simulink model "actividad3"  (R2021a)
settings: Solver=VariableStepAuto  StartTime=0.0  StopTime=2  FixedStep=1e-5  RelTol=1e-3
libraries: pid_lib x1
settings Model: Creator=Agus  LastModifiedBy=valen

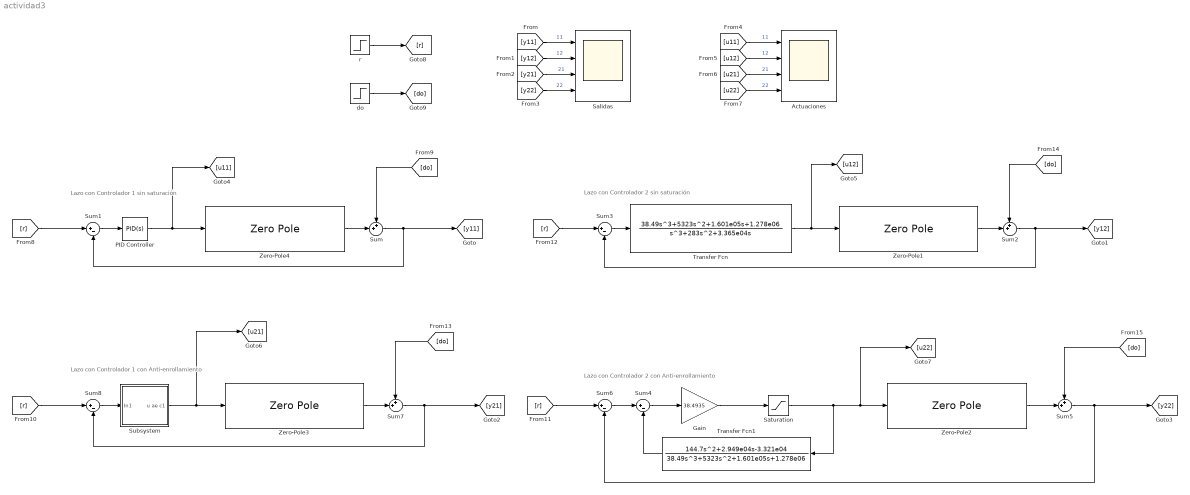
== system actividad3 ==
  note: Lazo con Controlador 1 con Anti-enrollamiento
  note: Lazo con Controlador 2 con Anti-enrollamiento
  note: Lazo con Controlador 1 sin saturación
  note: Lazo con Controlador 2 sin saturación
  Actuaciones : Scope  NumInputPorts=4
  Gain : Gain  Gain=38.4935
  PID Controller : pid_lib/PID Controller  Controller=PID  Form=Parallel  TimeDomain=Continuous-time  UseExternalTs=off  SampleTime=-1  IntegratorMethod=Forward Euler  FilterMethod=Forward Euler  ControllerParametersSource=internal  P=2.1595  I=8.175  D=0.0733  UseFilter=on  N=1364.25  TunerSelectOption=Transfer Function Based (PID Tuner App)  InitialConditionSource=internal  InitialConditionForIntegrator=0  InitialConditionForFilter=0  DifferentiatorICPrevScaledInput=0  ExternalReset=none  TrackingMode=off  Kt=1  LimitOutput=off  SatLimitsSource=internal  UpperSaturationLimit=inf  LowerSaturationLimit=-inf  LinearizeAsGain=on  AntiWindupMode=none  Kb=1  POutMin=[]  POutMax=[]  IOutMin=[]  IOutMax=[]  DOutMin=[]  DOutMax=[]  NOutMin=[]  NOutMax=[]  SumOutMin=[]  SumOutMax=[]  SaturationOutMin=[]  SaturationOutMax=[]  PParamMin=[]  PParamMax=[]  IParamMin=[]  IParamMax=[]  DParamMin=[]  DParamMax=[]  NParamMin=[]  NParamMax=[]  KbParamMin=[]  KbParamMax=[]  KtParamMin=[]  KtParamMax=[]  KbOutMin=[]  KbOutMax=[]  KtOutMin=[]  KtOutMax=[]  IntegratorOutMin=[]  IntegratorOutMax=[]  FilterOutMin=[]  FilterOutMax=[]  SumI1OutMin=[]  SumI1OutMax=[]  SumI2OutMin=[]  SumI2OutMax=[]  SumI3OutMin=[]  SumI3OutMax=[]  SumI4OutMin=[]  SumI4OutMax=[]  SumDOutMin=[]  SumDOutMax=[]  DifferentiatorOutMin=[]  DifferentiatorOutMax=[]  FilterDiffOutCoefMin=[]  FilterDiffOutCoefMax=[]  ReciprocalOutMin=[]  ReciprocalOutMax=[]  SumDenOutMin=[]  SumDenOutMax=[]  SumNumOutMin=[]  SumNumOutMax=[]  DivideOutMin=[]  DivideOutMax=[]  UdiffTsProdOutMin=[]  UdiffTsProdOutMax=[]  NTsProdOutMin=[]  NTsProdOutMax=[]  UintegralTsProdOutMin=[]  UintegralTsProdOutMax=[]  UngainTsProdOutMin=[]  UngainTsProdOutMax=[]  IntegratorContinuousStateAttributes=''  IntegratorStateMustResolveToSignalObject=off  IntegratorRTWStateStorageClass=Auto  FilterContinuousStateAttributes=''  FilterStateMustResolveToSignalObject=off  FilterRTWStateStorageClass=Auto  ParallelPVariant=InternalParameters  IdealPVariant=Disabled  IVariant=InternalParameters  DVariant=InternalParameters  IntegratorVariant=Continuous  SatVariant=Disabled  AWVariant=Passthrough  PCopyVariant=Disabled  TRVariant=Disabled  FdbkBlocksVariant=Forward  IdealPFdbkVariant=Disabled  SatFdbkVariant=Disabled  DerivativeFilterVariant=ContFilter  NVariant=InternalParameters  NCopyVariant=Disabled  FilterICVariant=InternalICsFilter  IntegratorICVariant=InternalICs  ExternalResetVariant=Disabled  TRSumVariant=Passthrough  SumFdbkVariant=Disabled  SumVariant=Sum_PID  TsampFilterVariant=InternalTs  TsampNgainVariant=Passthrough  TsampIntegralVariant=Passthrough  ExternalSaturationOutDataTypeStr=Inherit: Same as second input
  Salidas : Scope  NumInputPorts=4
  Saturation : Saturate  UpperLimit=7  LowerLimit=-7
  Subsystem : Subsystem  mask{Ki=8.175, Kp=2.1595, Kd=0.0733, tau=7.33e-4, sat=7}
  Sum{,2,5,7} (4 alike) : Sum  Inputs=++|
  Sum{1,3..4,6,8} (5 alike) : Sum  Inputs=|+-
  Transfer Fcn : TransferFcn  Numerator=[38.49 5323 1.601e05 1.278e06]  Denominator=[1 283 3.365e04 0]
  Transfer Fcn1 : TransferFcn  Numerator=[144.7 2.949e04 -3.321e04]  Denominator=[38.49 5323 1.601e05 1.278e06]
  Zero-Pole{1..4} (4 alike) : ZeroPole  Zeros=[]  Poles=[-100 -25 +25]  Gain=[57500]
  do : Step  SampleTime=0
  r : Step  Time=0  After=-1  SampleTime=0
  wires:
  PID Controller/1 -> Zero-Pole4/1, [u11]
  Zero-Pole4/1 -> Sum/2
  [do] -> Sum/1
  Sum1/1 -> PID Controller/1
  [r] -> Sum1/1
  Sum/1 -> [y11], Sum1/2
  Sum7/1 -> [y21], Sum8/2
  Transfer Fcn/1 -> Zero-Pole1/1, [u12]
  Sum2/1 -> [y12], Sum3/2
  Sum5/1 -> [y22], Sum6/2
  [do] -> Sum2/1
  Zero-Pole1/1 -> Sum2/2
  Saturation/1 -> Zero-Pole2/1, [u22], Transfer Fcn1/1
  [r] -> Sum3/1
  Sum3/1 -> Transfer Fcn/1
  Sum4/1 -> Gain/1
  [do] -> Sum5/1
  Transfer Fcn1/1 -> Sum4/2
  [r] -> Sum6/1
  Gain/1 -> Saturation/1
  Zero-Pole2/1 -> Sum5/2
  Sum6/1 -> Sum4/1
  [do] -> Sum7/1
  [r] -> Sum8/1
  Zero-Pole3/1 -> Sum7/2
  Subsystem/1(u ae c1) -> Zero-Pole3/1, [u21]
  Sum8/1 -> Subsystem/1(In1)
  [y11] -> Salidas/1  "11"
  [y12] -> Salidas/2  "12"
  [y21] -> Salidas/3  "21"
  [y22] -> Salidas/4  "22"
  [u11] -> Actuaciones/1  "11"
  [u12] -> Actuaciones/2  "12"
  [u21] -> Actuaciones/3  "21"
  [u22] -> Actuaciones/4  "22"
  r/1 -> [r]
  do/1 -> [do]

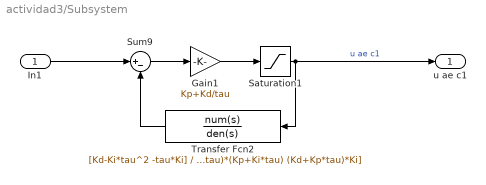
== system actividad3/Subsystem ==
  In1 : Inport
  Gain1 : Gain  Gain=Kp+Kd/tau
  Saturation1 : Saturate  UpperLimit=sat  LowerLimit=-sat
  Sum9 : Sum  Inputs=|+-
  Transfer Fcn2 : TransferFcn  Numerator=[Kd-Ki*tau^2 -tau*Ki]  Denominator=[(Kd+Kp*tau)^2 (Kd+Kp*tau)*(Kp+Ki*tau) (Kd+Kp*tau)*Ki]
  u ae c1 : Outport
  wires:
  Transfer Fcn2/1 -> Sum9/2
  Saturation1/1 -> u ae c1/1, Transfer Fcn2/1  "u ae c1"
  In1/1 -> Sum9/1
  Gain1/1 -> Saturation1/1
  Sum9/1 -> Gain1/1
